simulink model "temp_simulink"  (R2019a)
settings: Solver=VariableStepAuto  StartTime=0.0  StopTime=10.0  RelTol=1e-3
values from neighbouring files (symbols this model uses):
  k = 1    [temp_script_file.m]
  t_const = 1    [temp_script_file.m]
undefined symbols (not defined in the file or in its folder): K
settings Model: Creator=MahMoud  LastModifiedBy=MahMoud

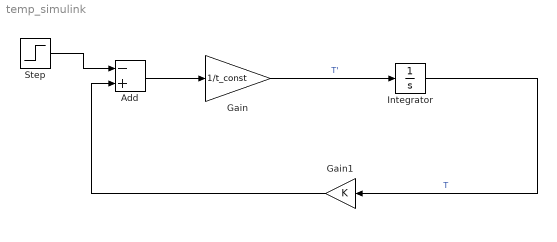
== system temp_simulink ==
  Add : Sum  Inputs=-+
  Gain : Gain  Gain=1/t_const
  Gain1 : Gain  Gain=K
  Integrator : Integrator
  Step : Step  After=1*k  SampleTime=0
  wires:
  Gain/1 -> Integrator/1  "T'"
  Add/1 -> Gain/1
  Integrator/1 -> Gain1/1  "T"
  Gain1/1 -> Add/2
  Step/1 -> Add/1
